simulink model "n_trotinettes_tout_discret"  (Simulink 6.5)
settings: Solver=ode45  StartTime=0.0  StopTime=stop+dt  RelTol=1e-6
values from neighbouring files (symbols this model uses):
  Af = -eye(3)/Tau    [lance_tout_propor.m]
  Bf = eye(N)/Tau    [lance_tout_propor.m]
  Cf = eye(N)    [lance_tout_propor.m]
  D = 0.01    [lance_tout.m]    (also in lance_tout_propor.m = 0.04254)
  Delta = (randn(N,1)*SDelta/100*NDelta)+NDelta    [lance_tout.m]    (also in lance_tout_propor.m)
  Df = zeros(N,N)    [lance_tout_propor.m]
  dt = 2    [lance_tout.m]    (also in lance_tout_propor.m)
  gama = vmax/dt    (= 1.5)    [lance_tout.m]    (also in lance_tout_propor.m = 1.65)
  Ka = Kry(:,N+1:N*2)    [lance_tout.m]    (also in lance_tout_propor.m)
  Ki = Kry(:,1:N)*(dim-2)    [lance_tout.m]    (also in lance_tout_propor.m = Kry(:,1:N))
  KphiSJv = (randn(N,1)*SKphiSJv/100*NKphiSJv)+NKphiSJv    [lance_tout.m]    (also in lance_tout_propor.m)
  Kpwm = (randn(N,1)*SKpwm/100*NKpwm)+NKpwm    [lance_tout.m]    (also in lance_tout_propor.m)
  Ktach = (randn(N,1)*SKtach/100*NKtach)+NKtach    [lance_tout.m]    (also in lance_tout_propor.m)
  Kv = Kry(:,N*2+1:3*N)    [lance_tout.m]    (also in lance_tout_propor.m)
  Ltrot = 1    [lance_tout_propor.m]
  M_ecart = 0    [lance_tout.m]    (also in lance_tout_propor.m)
  N = 3    [lance_tout.m]    (also in lance_tout_propor.m)
  NDelta = 4.254e-3    (= 0.004254)    [lance_tout.m]    (also in lance_tout_propor.m)
  NKtach = 2.5/3.33    (= 0.750750750751)    [lance_tout.m]    (also in lance_tout_propor.m)
  Si = (randn(N,1)*SSi/100*NSi)+NSi    [lance_tout.m]    (also in lance_tout_propor.m)
  start = 1    [lance_tout.m]    (also in lance_tout_propor.m)
  stop = start+10    (= 11)    [lance_tout.m]    (also in lance_tout_propor.m = 4.86727272727)
  Te = 2E-3    (= 0.002)    [lance_tout.m]    (also in lance_tout_propor.m)
  vmax = 3    [lance_tout.m]    (also in lance_tout_propor.m = 3.3)
undefined symbols (not defined in the file or in its folder): DiscIntNeverNeededParam
settings Model: Creator=admin  LastModifiedBy=admin
settings DataIOCC: SignalLoggingName=sigsOut
settings DebuggingCC: SolverPrmCheckMsg=none  MultiTaskDSMMsg=warning  MultiTaskCondExecSysMsg=none  StrictBusMsg=None
settings HardwareCC: TargetUnknown=on
settings RTWCC: IncludeERTFirstTime=on

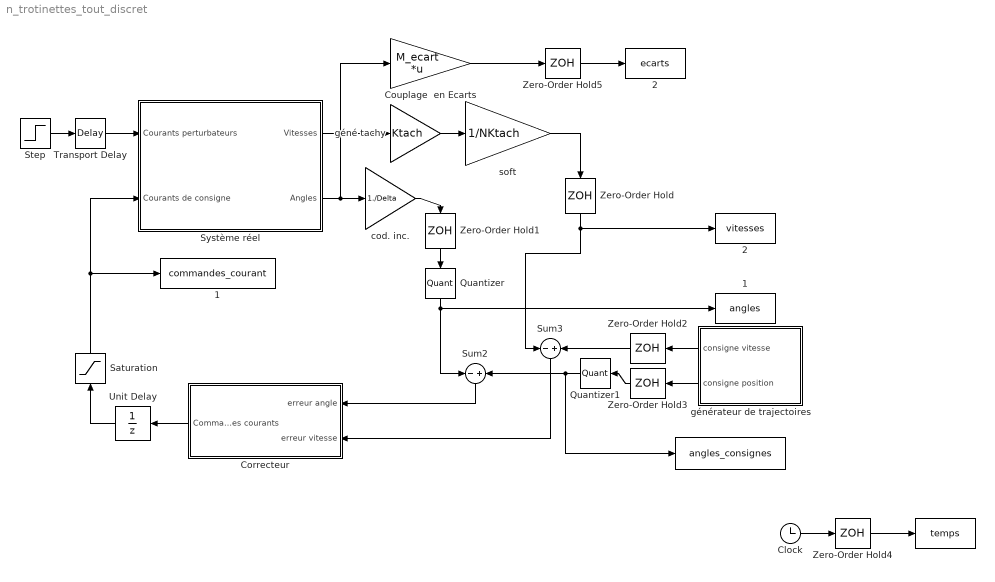
== system n_trotinettes_tout_discret ==
  " " : ToWorkspace  VariableName=temps  SampleTime=-1  SaveFormat=Array
  "  " : ToWorkspace  VariableName=angles_consignes  SampleTime=-1  SaveFormat=Array
  "   2" : ToWorkspace  VariableName=ecarts  SampleTime=-1  SaveFormat=Array
  "  1" : ToWorkspace  VariableName=angles  SampleTime=-1  SaveFormat=Array
  " 2" : ToWorkspace  VariableName=vitesses  SampleTime=-1  SaveFormat=Array
  "   1" : ToWorkspace  VariableName=commandes_courant  SampleTime=-1  SaveFormat=Array
  Clock : Clock
      settings: Decimation=10
  Correcteur : Subsystem  Orientation=left
  Couplage  en Ecarts : Gain  Gain=M_ecart  Multiplication=Matrix(K*u)  SaturateOnIntegerOverflow=on
  Quantizer : Quantizer  Orientation=down  QuantizationInterval=1
  Quantizer1 : Quantizer  Orientation=left  QuantizationInterval=1
  Saturation : Saturate  Orientation=up  UpperLimit=+1  LowerLimit=-1
  Step : Step  Time=(start+dt+0.1)  Before=zeros(N,1)  After=ones(N,1)*0  SampleTime=0
  Sum2 : Sum  Orientation=down  Inputs=-|+  SaturateOnIntegerOverflow=on
  Sum3 : Sum  Orientation=down  Inputs=-|+  SaturateOnIntegerOverflow=on
  Système réel : Subsystem
  Transport Delay : TransportDelay  DelayTime=(N-1)*(Ltrot+D)/vmax:-(Ltrot+D)/vmax:0  InitialOutput=zeros(N,1)
  Unit Delay : UnitDelay  Orientation=left  X0=zeros(N,1)  SampleTime=Te
  Zero-Order Hold : ZeroOrderHold  Orientation=down  SampleTime=Te
  Zero-Order Hold1 : ZeroOrderHold  Orientation=down  SampleTime=Te
  Zero-Order Hold2 : ZeroOrderHold  Orientation=left  SampleTime=Te
  Zero-Order Hold3 : ZeroOrderHold  Orientation=left  SampleTime=Te
  Zero-Order Hold4 : ZeroOrderHold  SampleTime=Te
  Zero-Order Hold5 : ZeroOrderHold  SampleTime=Te
  cod. inc. : Gain  Gain=1./Delta  SaturateOnIntegerOverflow=on
  géné tachy : Gain  Gain=Ktach  SaturateOnIntegerOverflow=on
  générateur de trajectoires : Subsystem  Orientation=left
  soft : Gain  Gain=1/NKtach  SaturateOnIntegerOverflow=on
  wires:
  Système réel/2(Angles) -> cod. inc./1, Couplage  en Ecarts/1
  générateur de trajectoires/2(consigne position) -> Zero-Order Hold3/1
  Clock/1 -> Zero-Order Hold4/1
  Correcteur/1(Commandes courants) -> Unit Delay/1
  Système réel/1(Vitesses) -> géné tachy/1
  Sum3/1 -> Correcteur/2(erreur vitesse)
  Sum2/1 -> Correcteur/1(erreur angle)
  générateur de trajectoires/1(consigne vitesse) -> Zero-Order Hold2/1
  Couplage  en Ecarts/1 -> Zero-Order Hold5/1
  géné tachy/1 -> soft/1
  cod. inc./1 -> Zero-Order Hold1/1
  Saturation/1 -> Système réel/2(Courants de consigne), "   1"/1
  soft/1 -> Zero-Order Hold/1
  Step/1 -> Transport Delay/1
  Transport Delay/1 -> Système réel/1(Courants perturbateurs)
  Zero-Order Hold/1 -> Sum3/1, " 2"/1
  Zero-Order Hold1/1 -> Quantizer/1
  Zero-Order Hold2/1 -> Sum3/2
  Zero-Order Hold3/1 -> Quantizer1/1
  Zero-Order Hold4/1 -> " "/1
  Quantizer/1 -> Sum2/1, "  1"/1
  Quantizer1/1 -> Sum2/2, "  "/1
  Unit Delay/1 -> Saturation/1
  Zero-Order Hold5/1 -> "   2"/1

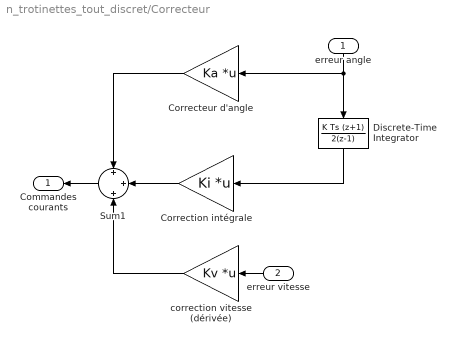
== system n_trotinettes_tout_discret/Correcteur ==
  erreur angle : Inport  Orientation=down
  erreur vitesse : Inport  Orientation=left  Port=2
  Correcteur d'angle : Gain  Orientation=left  Gain=Ka  Multiplication=Matrix(K*u)  SaturateOnIntegerOverflow=on
  Correction intégrale : Gain  Orientation=left  Gain=Ki  Multiplication=Matrix(K*u)  SaturateOnIntegerOverflow=on
  Discrete-Time Integrator : DiscreteIntegrator  Orientation=down  IntegratorMethod=Integration: Trapezoidal  SampleTime=Te  ICPrevOutput=DiscIntNeverNeededParam  ICPrevScaledInput=DiscIntNeverNeededParam
  Sum1 : Sum  Orientation=left  Inputs=+|+|+  SaturateOnIntegerOverflow=on  InputSameDT=on
  correction vitesse (dérivée) : Gain  Orientation=left  Gain=Kv  Multiplication=Matrix(K*u)  SaturateOnIntegerOverflow=on
  Commandes courants : Outport  Orientation=left
  wires:
  erreur angle/1 -> Correcteur d'angle/1, Discrete-Time Integrator/1
  Correcteur d'angle/1 -> Sum1/1
  Discrete-Time Integrator/1 -> Correction intégrale/1
  correction vitesse (dérivée)/1 -> Sum1/3
  Correction intégrale/1 -> Sum1/2
  Sum1/1 -> Commandes courants/1
  erreur vitesse/1 -> correction vitesse (dérivée)/1

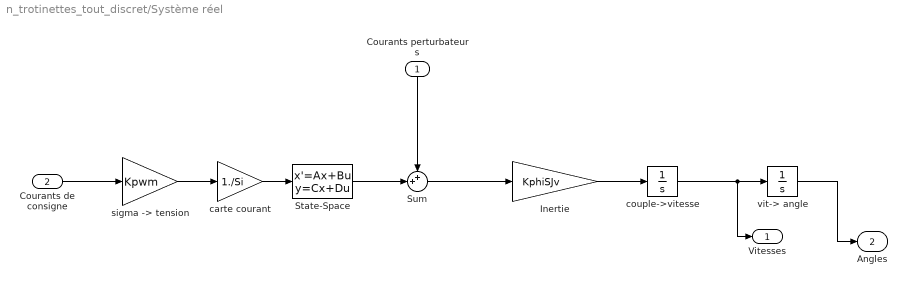
== system n_trotinettes_tout_discret/Système réel ==
  Courants perturbateurs : Inport  Orientation=down
  Courants de consigne : Inport  Port=2
  Inertie : Gain  Gain=KphiSJv  SaturateOnIntegerOverflow=on
  State-Space : StateSpace  A=Af  B=Bf  C=Cf  D=Df  X0=zeros(N,1)
  Sum : Sum  Inputs=++|  SaturateOnIntegerOverflow=on
  carte courant : Gain  Gain=1./Si  SaturateOnIntegerOverflow=on
  couple->vitesse : Integrator  InitialCondition=zeros(N,1)
  "sigma -> tension" : Gain  Gain=Kpwm  SaturateOnIntegerOverflow=on
  vit-> angle : Integrator  InitialCondition=(0:N-1)*D
  Vitesses : Outport
  Angles : Outport  Port=2
  wires:
  couple->vitesse/1 -> vit-> angle/1, Vitesses/1
  carte courant/1 -> State-Space/1
  Sum/1 -> Inertie/1
  vit-> angle/1 -> Angles/1
  Courants de consigne/1 -> "sigma -> tension"/1
  "sigma -> tension"/1 -> carte courant/1
  Inertie/1 -> couple->vitesse/1
  Courants perturbateurs/1 -> Sum/1
  State-Space/1 -> Sum/2

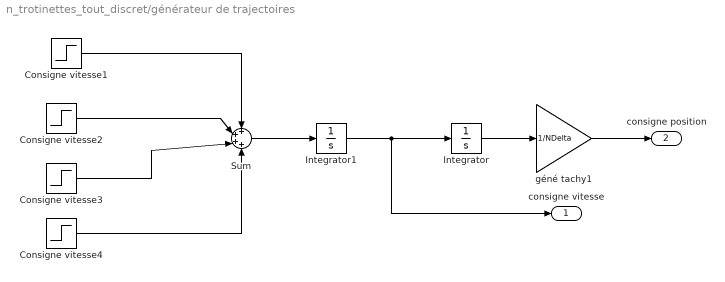
== system n_trotinettes_tout_discret/générateur de trajectoires ==
  Consigne vitesse1 : Step  Time=start  After=gama  SampleTime=0
  Consigne vitesse2 : Step  Time=start+dt  After=-gama  SampleTime=0
  Consigne vitesse3 : Step  Time=stop  After=-gama  SampleTime=0
  Consigne vitesse4 : Step  Time=stop+dt  After=gama  SampleTime=0
  Integrator : Integrator  InitialCondition=(0:(N-1))*D
  Integrator1 : Integrator  InitialCondition=zeros(N,1)
  Sum : Sum  Inputs=++++
  géné tachy1 : Gain  Gain=1/NDelta  SaturateOnIntegerOverflow=on
  consigne vitesse : Outport
  consigne position : Outport  Port=2
  wires:
  Integrator1/1 -> Integrator/1, consigne vitesse/1
  Integrator/1 -> géné tachy1/1
  géné tachy1/1 -> consigne position/1
  Consigne vitesse1/1 -> Sum/1
  Consigne vitesse2/1 -> Sum/2
  Consigne vitesse3/1 -> Sum/3
  Consigne vitesse4/1 -> Sum/4
  Sum/1 -> Integrator1/1
